simulink model "fxpdemo_multiword"  (Simulink 7.6)
settings: Solver=FixedStepDiscrete  StartTime=0.0  StopTime=1  FixedStep=1  RelTol=1e-3
libraries: rtwdemowidgets x1
Description:
  | Multi-Word Code Generation
  | 
  | This model demonstrates how wide integer and fixed-point operations are converted to multiword C code by Real-Time Workshop(R).
  | 
  | Multiword code is normally triggered by using parameters or signals with data types wider than C 'long'.
settings Model: Creator=The MathWorks Inc.  ExtModeAutoUpdateStatusClock=off
settings DataIOCC: LimitDataPoints=off
settings OptimizationCC: InitFltsAndDblsToZero=on  OptimizeModelRefInitCode=on  LifeSpan=1
settings DebuggingCC: SaveWithParameterizedLinksMsg=none  SignalResolutionControl=TryResolveAllWithWarning  StrictBusMsg=Warning
settings HardwareCC: ProdIntDivRoundTo=Zero  ProdEndianess=LittleEndian  ProdHWDeviceType=Specified  TargetEndianess=LittleEndian  TargetHWDeviceType=MATLAB Host
settings RTWCC: SystemTargetFile=ert.tlc  GenCodeOnly=on  TemplateMakefile=ert_default_tmf  Description=Real-Time Workshop Embedded Coder (no auto configuration)  GenerateReport=on  ProcessScript=ert_make_rtw_hook  IncludeHyperlinkInReport=on  LaunchReport=on
settings CodeAppCC: IgnoreCustomStorageClasses=off
settings ERTTargetCC: TargetFcnLib=ansi_tfl_tmw.mat  MultiwordLength=2048  GenerateSampleERTMain=on  InlinedParameterPlacement=NonHierarchical  ERTCustomFileTemplate=example_file_process.tlc  ConvertIfToSwitch=off

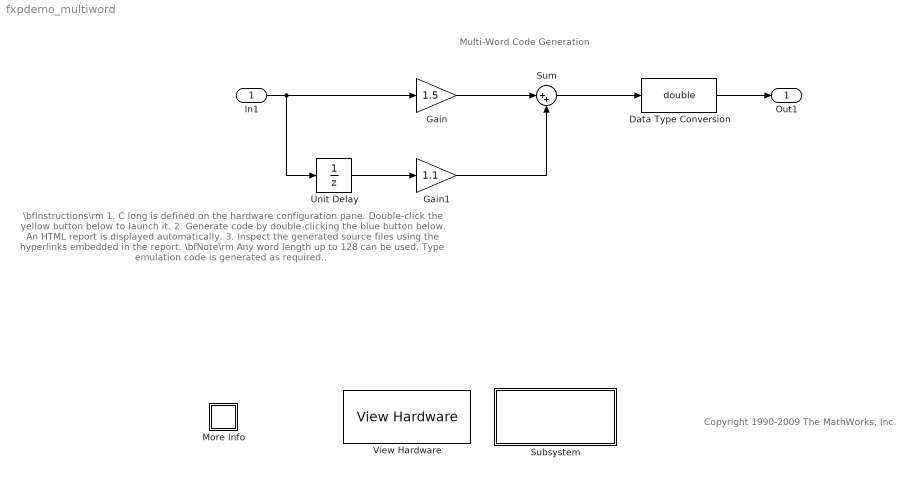
== system fxpdemo_multiword ==
  note: Copyright 1990-2009 The MathWorks, Inc.
  note: \bfInstructions\rm
      | 1. C long is defined on the hardware configuration pane. Double-click the yellow button
      |     below to launch it.
      | 2. Generate code by double-clicking the blue button below.
      |     An HTML report is displayed automatically.
      | 3. Inspect the generated source files using the hyperlinks embedded in the report.
      |
      | \bfNote\rm
      | Any word length up to 128 can be used. Type emulation code is generated as required..
  note: Multi-Word Code Generation
  In1 : Inport  OutDataTypeStr=fixdt(1,96,2^-3,0)
  Data Type Conversion : DataTypeConversion  OutDataTypeStr=double
  Gain : Gain  Gain=1.5  OutDataTypeStr=fixdt(1,128,20)  ParamDataTypeStr=Inherit: Same as input
  Gain1 : Gain  Gain=1.1  OutDataTypeStr=fixdt(1,128,20)
  More Info : Subsystem
      settings: OpenFcn=showdemo(bdroot(gcs))
      mask Display: disp('?')
  Subsystem : Subsystem
      settings: OpenFcn=rtwbuilddemomodel(bdroot);
      mask Display: disp('Generate Code\n(double-click)')
  Sum : Sum  Inputs=|++
  Unit Delay : UnitDelay  SampleTime=-1
  View Hardware : rtwdemowidgets/View Hardware  SystemSampleTime=-1
  Out1 : Outport
  wires:
  In1/1 -> Gain/1, Unit Delay/1
  Unit Delay/1 -> Gain1/1
  Gain/1 -> Sum/1
  Gain1/1 -> Sum/2
  Sum/1 -> Data Type Conversion/1
  Data Type Conversion/1 -> Out1/1

== system fxpdemo_multiword/More Info ==

== system fxpdemo_multiword/Subsystem ==
